simulink model "MotorCC_Simulacao"  (Simulink 8.1)
settings: Solver=ode45  StartTime=0.0  StopTime=2.5  RelTol=1e-3
values from neighbouring files (symbols this model uses):
  A = [0.960706073539 0.0654898774344 -0.385928713202 0.643214522003 0.0392939264606 0.934510122566 0.385928713202 -0.643214522003 0.197361633725 0.00439727712447 0.960706073539 0.0654898774344 ... (16 elements, 4x4)]    [Copy_of_ochi_inf.mat]    (also in MotorCC.m = [-120.5 1; -560 0]; aula11lmiyalmip.m = [1 1;0 2]; aula3.m = Sys.A; aula4.m = Sys.A)
  B = [0.00397352224227 4.41295962101e-05 0.0394723267451 0.000879455424894]    [Copy_of_ochi_inf.mat]    (also in MotorCC.m = [0 ; 500]; aula11lmiyalmip.m = [0;1]; aula3.m = Sys.B; aula4.m = Sys.B)
  C = [0 1 0 0]    [Copy_of_ochi_inf.mat]    (also in MotorCC.m = [1 0]; aula3.m = [1 0]; aula4.m; aula7dlqrcon.m = [1 0])
  D = [0]    [MotorCC.m]
  q0 = inv(K)*v0'    [MotorCC.m]
settings Model: Creator=hector  LastModifiedBy=hector

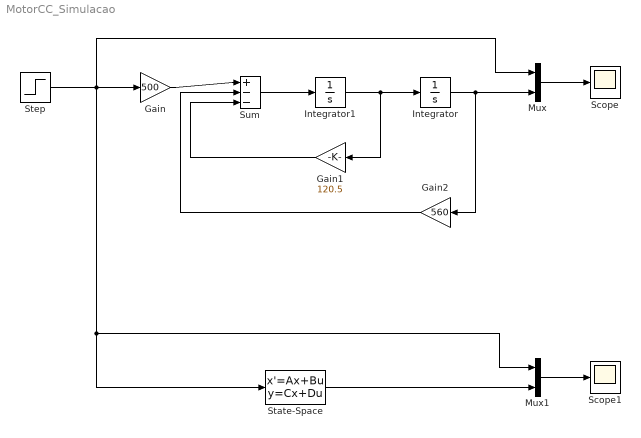
== system MotorCC_Simulacao ==
  Gain : Gain  Gain=500
  Gain1 : Gain  Gain=120.5
  Gain2 : Gain  Gain=560
  Integrator : Integrator  InitialCondition=1
  Integrator1 : Integrator  InitialCondition=2
  Mux : Mux  Inputs=2
  Mux1 : Mux  Inputs=2
  Scope : Scope
  Scope1 : Scope
  State-Space : StateSpace  A=A  B=B  C=C  D=D  X0=q0
  Step : Step  Time=0  SampleTime=0
  Sum : Sum  Inputs=|+--
  wires:
  Sum/1 -> Integrator1/1
  Integrator1/1 -> Integrator/1, Gain1/1
  Step/1 -> Gain/1, Mux/1, State-Space/1, Mux1/1
  Integrator/1 -> Gain2/1, Mux/2
  Gain1/1 -> Sum/3
  Gain2/1 -> Sum/2
  Mux/1 -> Scope/1
  Gain/1 -> Sum/1
  Mux1/1 -> Scope1/1
  State-Space/1 -> Mux1/2
